simulink model "Q_3_2_a"  (R2023b)
settings: Solver=VariableStepAuto  StartTime=0.0  StopTime=400e-3  MaxStep=tstepMax  RelTol=1e-3
undefined symbols (not defined in the file or in its folder): v_in
libraries: spsDiodeLib x12, spsSeriesRLCBranchLib x12, spsCurrentMeasurementLib x4, spsACVoltageSourceLib x3, spsVoltageMeasurementLib x2, spspowerguiLib x1
settings Model: Creator=abdulkadir  LastModifiedBy=abdulkadir
settings DataIOCC: ReturnWorkspaceOutputs=off

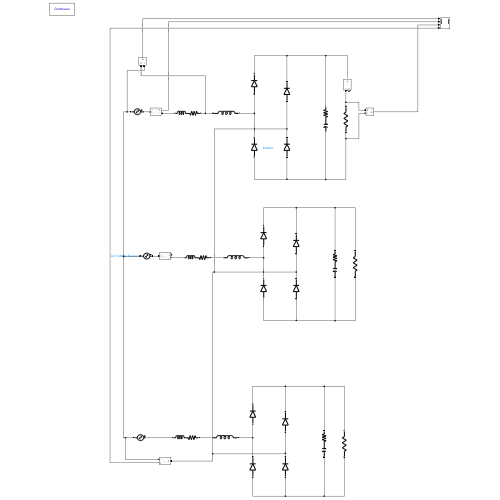
[thumbnail: Simulink's stored preview of the top-level diagram]
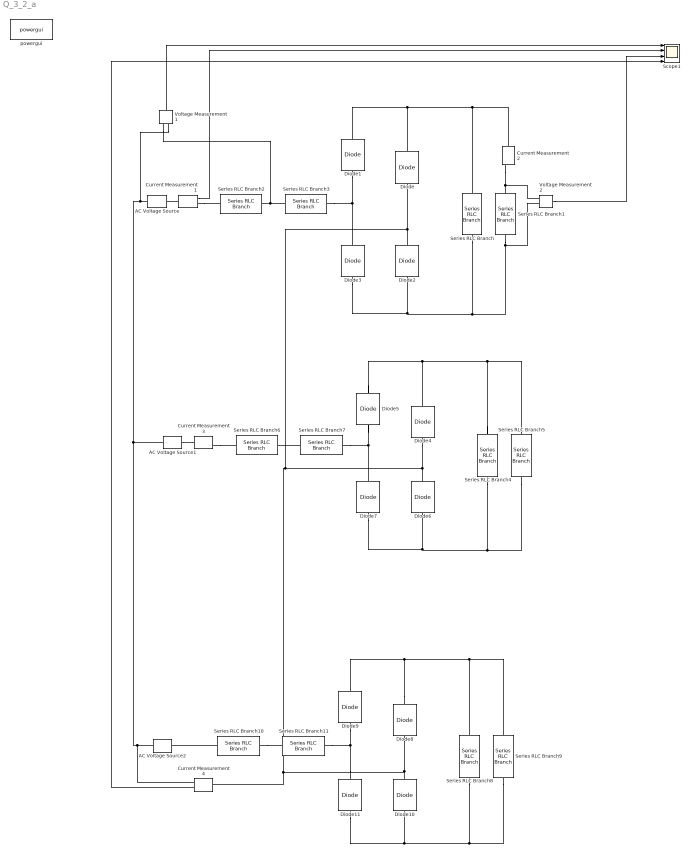
== system Q_3_2_a ==
  AC Voltage Source : spsACVoltageSourceLib/AC Voltage Source  Amplitude=v_in  Phase=0  Frequency=50  SampleTime=0  Measurements=None  BusType=swing  Pref=10e3  Qref=0  Qmin=-inf  Qmax=+inf
  AC Voltage Source1 : spsACVoltageSourceLib/AC Voltage Source  Amplitude=v_in  Phase=120  Frequency=50  SampleTime=0  Measurements=None  BusType=swing  Pref=10e3  Qref=0  Qmin=-inf  Qmax=+inf
  AC Voltage Source2 : spsACVoltageSourceLib/AC Voltage Source  Amplitude=v_in  Phase=240  Frequency=50  SampleTime=0  Measurements=None  BusType=swing  Pref=10e3  Qref=0  Qmin=-inf  Qmax=+inf
  Current Measurement{1..4} (4 alike) : spsCurrentMeasurementLib/Current Measurement  PhasorSimulation=off  OutputType=Complex  PSBequivalent=0
  Diode{,1..11} (12 alike) : spsDiodeLib/Diode  Ron=0  Lon=0  Vf=0  IC=0  UseSnubber=0  Rs=0  Cs=0  Measurements=off
  Scope1 : Scope  NumInputPorts=4
  Series RLC Branch : spsSeriesRLCBranchLib/Series RLC Branch  LConnTagsString=__new0  RConnTagsString=__new0  BranchType=RC  Resistance=1e-3  Inductance=1e-3  SetiL0=off  InitialCurrent=0  Capacitance=470e-6  Setx0=off  InitialVoltage=0  Measurements=None
  Series RLC Branch1 : spsSeriesRLCBranchLib/Series RLC Branch  LConnTagsString=__new0  RConnTagsString=__new0  BranchType=R  Resistance=60  Inductance=1e-3  SetiL0=off  InitialCurrent=0  Capacitance=470e-6  Setx0=off  InitialVoltage=0  Measurements=None
  Series RLC Branch10 : spsSeriesRLCBranchLib/Series RLC Branch  LConnTagsString=__new0  RConnTagsString=__new0  BranchType=RL  Resistance=0.1  Inductance=0.28e-3  SetiL0=off  InitialCurrent=0  Capacitance=470e-6  Setx0=off  InitialVoltage=0  Measurements=None
  Series RLC Branch11 : spsSeriesRLCBranchLib/Series RLC Branch  LConnTagsString=__new0  RConnTagsString=__new0  BranchType=L  Resistance=0.1  Inductance=3e-3  SetiL0=off  InitialCurrent=0  Capacitance=470e-6  Setx0=off  InitialVoltage=0  Measurements=None
  Series RLC Branch2 : spsSeriesRLCBranchLib/Series RLC Branch  LConnTagsString=__new0  RConnTagsString=__new0  BranchType=RL  Resistance=0.1  Inductance=0.28e-3  SetiL0=off  InitialCurrent=0  Capacitance=470e-6  Setx0=off  InitialVoltage=0  Measurements=None
  Series RLC Branch3 : spsSeriesRLCBranchLib/Series RLC Branch  LConnTagsString=__new0  RConnTagsString=__new0  BranchType=L  Resistance=0.1  Inductance=3e-3  SetiL0=off  InitialCurrent=0  Capacitance=470e-6  Setx0=off  InitialVoltage=0  Measurements=None
  Series RLC Branch4 : spsSeriesRLCBranchLib/Series RLC Branch  LConnTagsString=__new0  RConnTagsString=__new0  BranchType=RC  Resistance=1e-3  Inductance=1e-3  SetiL0=off  InitialCurrent=0  Capacitance=470e-6  Setx0=off  InitialVoltage=0  Measurements=None
  Series RLC Branch5 : spsSeriesRLCBranchLib/Series RLC Branch  LConnTagsString=__new0  RConnTagsString=__new0  BranchType=R  Resistance=60  Inductance=1e-3  SetiL0=off  InitialCurrent=0  Capacitance=470e-6  Setx0=off  InitialVoltage=0  Measurements=None
  Series RLC Branch6 : spsSeriesRLCBranchLib/Series RLC Branch  LConnTagsString=__new0  RConnTagsString=__new0  BranchType=RL  Resistance=0.1  Inductance=0.28e-3  SetiL0=off  InitialCurrent=0  Capacitance=470e-6  Setx0=off  InitialVoltage=0  Measurements=None
  Series RLC Branch7 : spsSeriesRLCBranchLib/Series RLC Branch  LConnTagsString=__new0  RConnTagsString=__new0  BranchType=L  Resistance=0.1  Inductance=3e-3  SetiL0=off  InitialCurrent=0  Capacitance=470e-6  Setx0=off  InitialVoltage=0  Measurements=None
  Series RLC Branch8 : spsSeriesRLCBranchLib/Series RLC Branch  LConnTagsString=__new0  RConnTagsString=__new0  BranchType=RC  Resistance=1e-3  Inductance=1e-3  SetiL0=off  InitialCurrent=0  Capacitance=470e-6  Setx0=off  InitialVoltage=0  Measurements=None
  Series RLC Branch9 : spsSeriesRLCBranchLib/Series RLC Branch  LConnTagsString=__new0  RConnTagsString=__new0  BranchType=R  Resistance=60  Inductance=1e-3  SetiL0=off  InitialCurrent=0  Capacitance=470e-6  Setx0=off  InitialVoltage=0  Measurements=None
  Voltage Measurement1 : spsVoltageMeasurementLib/Voltage Measurement  PhasorSimulation=off  OutputType=Complex  PSBequivalent=0
  Voltage Measurement2 : spsVoltageMeasurementLib/Voltage Measurement  PhasorSimulation=off  OutputType=Complex  PSBequivalent=0
  powergui : spspowerguiLib/powergui  Priority=1  SimulationMode=Continuous  SampleTime=0.1e-3  frequency=60  Iterations=50  frequencyindice=50  Pbase=100e6  ErrMax=1e-4  UnitsV=kV  UnitsW=MW  buscounter=0  FunctionMessages=off  echomessages=off  EnableUseOfTLC=off  CurrentSourceSwitches=off  DisableSnubberDevices=off  DisableRonSwitches=off  DisableVfSwitches=off  DisplayEquations=off  AutomaticDiscreteSolvers=off  SolverType=Tustin/Backward Euler (TBE)  Interpol=off  ExternalGateDelay=off  methode=off  Ts=100  x0status=blocks  SPID=on  SwTol=0  HookPort=off  NonlinearTolerance=1e-4  nMaxIteration=100  ContinueOnMaxIteration=off  RestoreLinks=warning  ResistiveCurrentMeasurement=off  Frange=[0:2:500]  Ylog=off  Xlog=on  ShowGrid=off  save=off  variable=ZData  structure=0  ZoomFFT=off  StartTime=0.0  cycles=1  DisplayStyle=1  fundamental=60  FreqAxis=off  MaxFrequency=1000  frequencyindicesteady=1  RmsSteady=1  display=off
  wires:
  Current Measurement1/1 -> Scope1/2
  Voltage Measurement2/1 -> Scope1/3
  Voltage Measurement1/1 -> Scope1/1
  Current Measurement4/1 -> Scope1/4
  connections:
  Series RLC Branch/LConn1 -- Current Measurement2/LConn1 -- Diode1/RConn1 -- Diode/RConn1
  Series RLC Branch/RConn1 -- Voltage Measurement2/LConn2 -- Series RLC Branch1/RConn1 -- Diode3/LConn1 -- Diode2/LConn1
  Current Measurement1/LConn1 -- AC Voltage Source/RConn1
  Diode1/LConn1 -- Series RLC Branch3/LConn1 -- Diode3/RConn1
  Current Measurement2/RConn1 -- Voltage Measurement2/LConn1 -- Series RLC Branch1/LConn1
  Current Measurement1/RConn1 -- Series RLC Branch2/RConn1
  Series RLC Branch2/LConn1 -- Voltage Measurement1/LConn1 -- Series RLC Branch3/RConn1
  Series RLC Branch4/RConn1 -- Series RLC Branch5/RConn1 -- Diode7/LConn1 -- Diode6/LConn1
  Diode5/LConn1 -- Diode7/RConn1 -- Series RLC Branch7/LConn1
  Series RLC Branch4/LConn1 -- Series RLC Branch5/LConn1 -- Diode4/RConn1 -- Diode5/RConn1
  Series RLC Branch6/LConn1 -- Series RLC Branch7/RConn1
  Current Measurement3/RConn1 -- Series RLC Branch6/RConn1
  Current Measurement3/LConn1 -- AC Voltage Source1/RConn1
  Series RLC Branch9/RConn1 -- Series RLC Branch8/RConn1 -- Diode10/LConn1 -- Diode11/LConn1
  Diode11/RConn1 -- Diode9/LConn1 -- Series RLC Branch11/LConn1
  Diode8/RConn1 -- Series RLC Branch9/LConn1 -- Series RLC Branch8/LConn1 -- Diode9/RConn1
  Series RLC Branch10/LConn1 -- Series RLC Branch11/RConn1
  Series RLC Branch10/RConn1 -- AC Voltage Source2/RConn1
  Diode2/RConn1 -- Current Measurement4/LConn1 -- Diode8/LConn1 -- Diode10/RConn1 -- Diode4/LConn1 -- Diode6/RConn1 -- Diode/LConn1
  AC Voltage Source2/LConn1 -- Current Measurement4/RConn1 -- Voltage Measurement1/LConn2 -- AC Voltage Source/LConn1 -- AC Voltage Source1/LConn1
